simulink model "dynamic_model_2015"  (R2015b)
settings: Solver=FixedStepAuto  StartTime=0.0  StopTime=sim_time  FixedStep=0.01  RelTol=1e-3
values from neighbouring files (symbols this model uses):
  b = 0.75    [d_model_sig.m]    (also in d_model_sim.m; modelo_cinematico.m = 2; untitled.mat = 1)
  B = 0.0001    [d_model_sig.m]    (also in d_model_sim.m = 0.001)
  D = 33    [d_model_sig.m]    (also in d_model_sim.m)
  J = 17.3175    [d_model_sig.m]    (also in d_model_sim.m)
  mc = 30    [d_model_sig.m]    (also in d_model_sim.m)
  r = 0.1    [d_model_sig.m]    (also in d_model_sim.m; untitled.mat = 1)
  s = 0.3    [d_model_sig.m]    (also in d_model_sim.m)
  theta0 = 0    [d_model_sim.m]
  v0 = 0    [d_model_sim.m]
  w0 = 0    [d_model_sim.m]
  x0 = 0    [d_model_sim.m]
  y0 = 0    [d_model_sim.m]
settings Model: Creator=estebanza  LastModifiedBy=estebanza
settings DataIOCC: LimitDataPoints=off
settings DebuggingCC: AllowSymbolicDim=on
settings ModelReferenceCC: PropagateSignalLabelsOutOfModel=on
settings GRTTargetCC: GeneratePreprocessorConditionals=Disable all

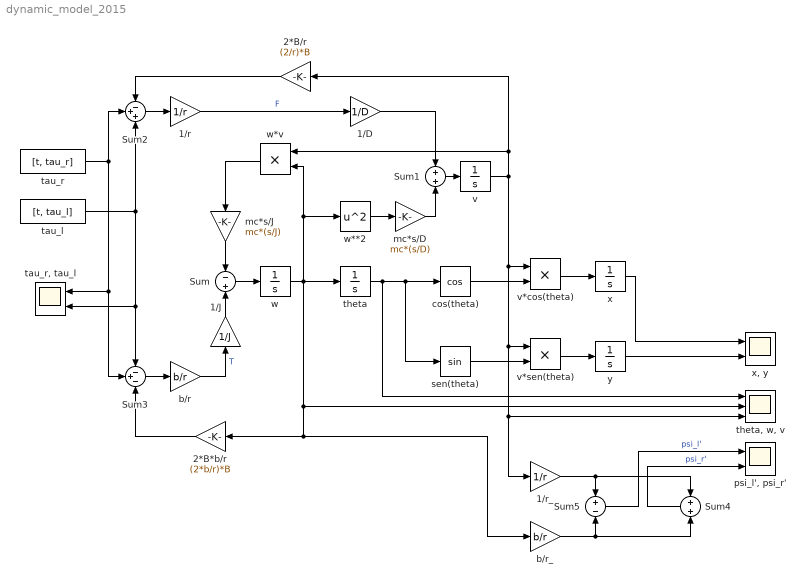
== system dynamic_model_2015 ==
  1/D : Gain  Gain=1/D
  1/J : Gain  Gain=1/J
  1/r : Gain  Gain=1/r
  1/r_ : Gain  Gain=1/r
  2*B*b/r : Gain  Gain=(2*b/r)*B
  2*B/r : Gain  Gain=(2/r)*B
  Sum : Sum  Inputs=-+
  Sum1 : Sum
  Sum2 : Sum  Inputs=-++
  Sum3 : Sum  Inputs=-+-
  Sum4 : Sum  Inputs=+|+
  Sum5 : Sum  Inputs=+|-
  b/r : Gain  Gain=b/r
  b/r_ : Gain  Gain=b/r
  cos(theta) : Trigonometry  Operator=cos
  mc*s/D : Gain  Gain=mc*(s/D)
  mc*s/J : Gain  Gain=mc*(s/J)
  "psi_l', psi_r'" : Scope  NumInputPorts=2
  sen(theta) : Trigonometry
  tau_l : FromWorkspace  VariableName=[t, tau_l]  SampleTime=0  OutputAfterFinalValue=Setting to zero
  tau_r : FromWorkspace  VariableName=[t, tau_r]  SampleTime=0  OutputAfterFinalValue=Setting to zero
  "tau_r, tau_l" : Scope  NumInputPorts=2
  theta : Integrator  InitialCondition=theta0
  "theta, w, v" : Scope  NumInputPorts=3
  v : Integrator  InitialCondition=v0
  v*cos(theta) : Product
  v*sen(theta) : Product
  w : Integrator  InitialCondition=w0
  w**2 : Math  Operator=square  SaturateOnIntegerOverflow=on
  w*v : Product
  x : Integrator  InitialCondition=x0
  "x, y" : Scope  NumInputPorts=2
  y : Integrator  InitialCondition=y0
  wires:
  v*cos(theta)/1 -> x/1
  cos(theta)/1 -> v*cos(theta)/2
  theta/1 -> sen(theta)/1, cos(theta)/1, "theta, w, v"/1
  Sum/1 -> w/1
  w/1 -> w**2/1, w*v/2, b/r_/1, 2*B*b/r/1, "theta, w, v"/2, theta/1
  1/J/1 -> Sum/2
  mc*s/J/1 -> Sum/1
  w*v/1 -> mc*s/J/1
  v*sen(theta)/1 -> y/1
  sen(theta)/1 -> v*sen(theta)/2
  b/r/1 -> 1/J/1  "T"
  Sum1/1 -> v/1
  w**2/1 -> mc*s/D/1
  1/D/1 -> Sum1/1
  1/r/1 -> 1/D/1  "F"
  Sum2/1 -> 1/r/1
  Sum3/1 -> b/r/1
  tau_l/1 -> Sum3/1, "tau_r, tau_l"/2, Sum2/3
  x/1 -> "x, y"/1
  y/1 -> "x, y"/2
  v/1 -> 1/r_/1, "theta, w, v"/3, v*sen(theta)/1, v*cos(theta)/1, 2*B/r/1, w*v/1
  b/r_/1 -> Sum4/2, Sum5/2
  1/r_/1 -> Sum4/1, Sum5/1
  Sum5/1 -> "psi_l', psi_r'"/1  "psi_l'"
  Sum4/1 -> "psi_l', psi_r'"/2  "psi_r'"
  2*B/r/1 -> Sum2/1
  2*B*b/r/1 -> Sum3/3
  mc*s/D/1 -> Sum1/2
  tau_r/1 -> "tau_r, tau_l"/1, Sum3/2, Sum2/2
